simulink model "reference_signal_in_time"  (R2021a)
settings: Solver=VariableStepAuto  StartTime=0.0  StopTime=time_traj(N)+5  RelTol=1e-3
values from neighbouring files (symbols this model uses):
  b = 2    [main_script.m]    (also in trilat2.m = dhat.^2-beacons(:,1).^2-beacons(:,2).^2)
  k1 = 0.5    [main_script.m]
  k1_r = 1    [main_script.m]
  k2 = 1    [main_script.m]
  k2_r = 10    [main_script.m]
  k3_r = 10    [main_script.m]
  N = length(time_traj)    [main_script.m]    (also in trilat2.m = size(beacons,1))
  P0 = diag([0.15 0.15 deg2rad(10)].^2)    [main_script.m]
  S = [  0  100 ... (first row only)    [main_script.m]
  t_sw = time_traj(N-1)+((time_traj(N)-time_traj(N-1))*8/10)    [main_script.m]
  theta0 = 0.001    [main_script.m]
  V = eye(3)*0.01^2    [main_script.m]
  W = 10*diag([1 1 deg2rad(5)].^2)    [main_script.m]
  x0 = x0_g(1,1)+10    [main_script.m]
  x0_g = ginput    [enviroment_plot.m]    (also in main_script.m = enviroment_plot(axis_enviroment))
  y0 = x0_g(1,2)-10    [main_script.m]
libraries: simulink x4, robotcorelib x2
settings Model: Creator=csanc  LastModifiedBy=csanc

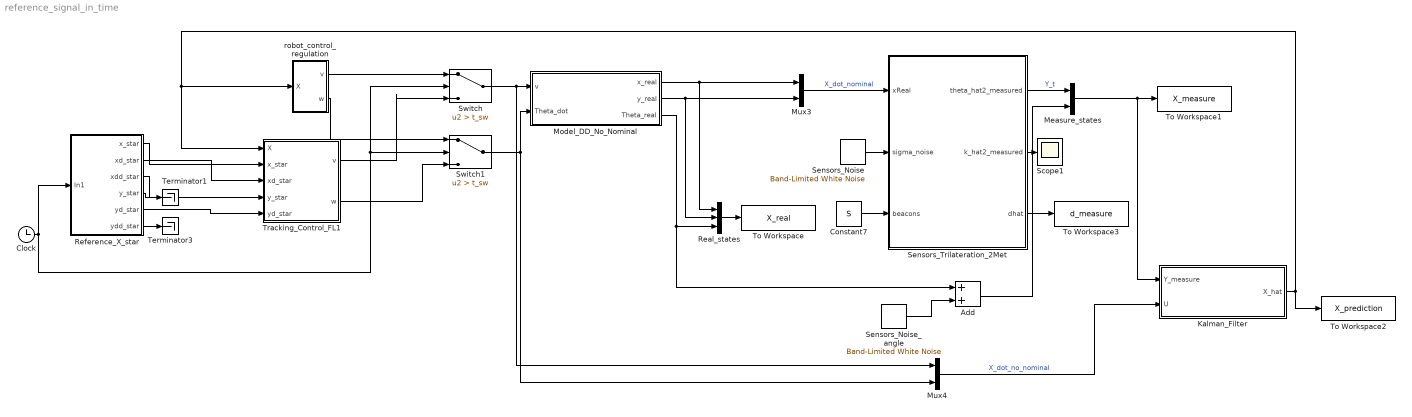
== system reference_signal_in_time ==
  Add : Sum
  Clock : Clock
  Constant7 : Constant  Value=S
  Kalman_Filter : Subsystem
  Measure_states : Mux  Inputs=2
  Model_DD_No_Nominal : Subsystem
  Mux3 : Mux  Inputs=2
  Mux4 : Mux  Inputs=2
  Real_states : Mux  Inputs=3
  Reference_X_star : Subsystem
  Scope1 : Scope
  Sensors_Noise : simulink/Sources/Band-Limited White Noise  Cov=[0.08]  Ts=0.05  seed=[23341]
  Sensors_Noise_angle : simulink/Sources/Band-Limited White Noise  Cov=[0.001]  Ts=0.05  seed=[23341]
  Sensors_Trilateration_2Met : MATLAB Function  TreatAsAtomicUnit=on
  Switch : Switch  Criteria=u2 > Threshold  Threshold=t_sw
  Switch1 : Switch  Criteria=u2 > Threshold  Threshold=t_sw
  Terminator1 : Terminator
  Terminator3 : Terminator
  To Workspace : ToWorkspace  VariableName=X_real  SaveFormat=Structure  SampleTime=-1
  To Workspace1 : ToWorkspace  VariableName=X_measure  SaveFormat=Structure  SampleTime=-1
  To Workspace2 : ToWorkspace  VariableName=X_prediction  SaveFormat=Structure  SampleTime=-1
  To Workspace3 : ToWorkspace  VariableName=d_measure  SaveFormat=Structure  SampleTime=-1
  Tracking_Control_FL1 : Subsystem
  robot_control_regulation : Subsystem
  wires:
  Clock/1 -> Reference_X_star/1(In1), Switch1/2, Switch/2
  Mux4/1 -> Kalman_Filter/2(U)  "X_dot_no_nominal"
  Model_DD_No_Nominal/2(y_real) -> Real_states/2, Mux3/2
  Sensors_Trilateration_2Met/1(theta_hat2_measured) -> Measure_states/1  "Y_t"
  Constant7/1 -> Sensors_Trilateration_2Met/3(beacons)
  Mux3/1 -> Sensors_Trilateration_2Met/1(xReal)  "X_dot_nominal"
  Sensors_Noise/1 -> Sensors_Trilateration_2Met/2(sigma_noise)
  Sensors_Trilateration_2Met/2(k_hat2_measured) -> Scope1/1
  Measure_states/1 -> To Workspace1/1, Kalman_Filter/1(Y_measure)
  Model_DD_No_Nominal/1(x_real) -> Real_states/1, Mux3/1
  Switch/1 -> Mux4/1, Model_DD_No_Nominal/1(v)
  Switch1/1 -> Model_DD_No_Nominal/2(Theta_dot), Mux4/2
  Model_DD_No_Nominal/3(Theta_real) -> Add/1, Real_states/3
  Reference_X_star/3(xdd_star) -> Terminator1/1
  Reference_X_star/6(ydd_star) -> Terminator3/1
  Real_states/1 -> To Workspace/1
  Kalman_Filter/1(X_hat) -> Tracking_Control_FL1/1(X), robot_control_regulation/1(X), To Workspace2/1
  Sensors_Trilateration_2Met/3(dhat) -> To Workspace3/1
  Sensors_Noise_angle/1 -> Add/2
  Add/1 -> Measure_states/2
  robot_control_regulation/1(v) -> Switch/1
  robot_control_regulation/2(w) -> Switch1/1
  Reference_X_star/1(x_star) -> Tracking_Control_FL1/2(x_star)
  Reference_X_star/2(xd_star) -> Tracking_Control_FL1/3(xd_star)
  Reference_X_star/4(y_star) -> Tracking_Control_FL1/4(y_star)
  Reference_X_star/5(yd_star) -> Tracking_Control_FL1/5(yd_star)
  Tracking_Control_FL1/1(v) -> Switch/3
  Tracking_Control_FL1/2(w) -> Switch1/3

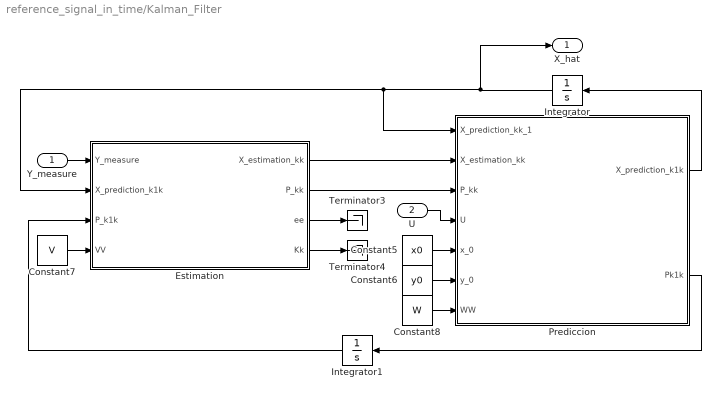
== system reference_signal_in_time/Kalman_Filter ==
  Y_measure : Inport
  U : Inport  Port=2
  Constant5 : Constant  Value=x0
  Constant6 : Constant  Value=y0
  Constant7 : Constant  Value=V
  Constant8 : Constant  Value=W
  Estimation : MATLAB Function  TreatAsAtomicUnit=on
  Integrator : Integrator  InitialCondition=[x0;y0;theta0]
  Integrator1 : Integrator  InitialCondition=P0
  Prediccion : MATLAB Function  TreatAsAtomicUnit=on
  Terminator3 : Terminator
  Terminator4 : Terminator
  X_hat : Outport
  wires:
  Estimation/3(ee) -> Terminator3/1
  Integrator/1 -> X_hat/1, Prediccion/1(X_prediction_kk_1), Estimation/2(X_prediction_k1k)
  Estimation/4(Kk) -> Terminator4/1
  Constant7/1 -> Estimation/4(VV)
  Constant5/1 -> Prediccion/5(x_0)
  Integrator1/1 -> Estimation/3(P_k1k)
  Y_measure/1 -> Estimation/1(Y_measure)
  Constant6/1 -> Prediccion/6(y_0)
  Prediccion/1(X_prediction_k1k) -> Integrator/1
  Prediccion/2(Pk1k) -> Integrator1/1
  Constant8/1 -> Prediccion/7(WW)
  Estimation/1(X_estimation_kk) -> Prediccion/2(X_estimation_kk)
  U/1 -> Prediccion/4(U)
  Estimation/2(P_kk) -> Prediccion/3(P_kk)

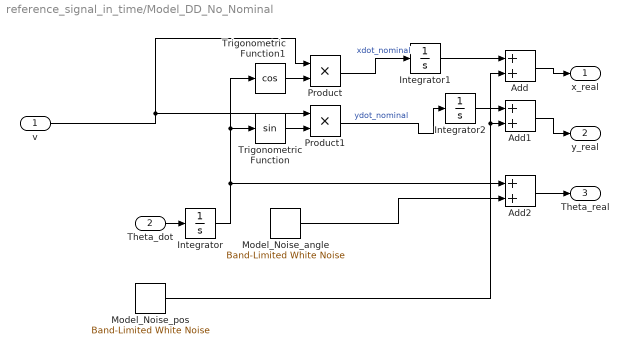
== system reference_signal_in_time/Model_DD_No_Nominal ==
  v : Inport
  Theta_dot : Inport  Port=2
  Add : Sum
  Add1 : Sum
  Add2 : Sum
  Integrator : Integrator  InitialCondition=theta0
  Integrator1 : Integrator  InitialCondition=x0
  Integrator2 : Integrator  InitialCondition=y0
  Model_Noise_angle : simulink/Sources/Band-Limited White Noise  Cov=[0.0001]  Ts=0.05  seed=[23341]
  Model_Noise_pos : simulink/Sources/Band-Limited White Noise  Cov=[0.001]  Ts=0.05  seed=[23341]
  Product : Product
  Product1 : Product
  Trigonometric Function : Trigonometry
  Trigonometric Function1 : Trigonometry  Operator=cos
  x_real : Outport
  y_real : Outport  Port=2
  Theta_real : Outport  Port=3
  wires:
  Theta_dot/1 -> Integrator/1
  Trigonometric Function/1 -> Product1/2
  Product1/1 -> Integrator2/1  "ydot_nominal"
  Trigonometric Function1/1 -> Product/2
  Integrator/1 -> Add2/1, Trigonometric Function/1, Trigonometric Function1/1
  v/1 -> Product/1, Product1/1
  Product/1 -> Integrator1/1  "xdot_nominal"
  Integrator1/1 -> Add/1
  Add/1 -> x_real/1
  Integrator2/1 -> Add1/1
  Add1/1 -> y_real/1
  Add2/1 -> Theta_real/1
  Model_Noise_pos/1 -> Add1/2, Add/2
  Model_Noise_angle/1 -> Add2/2

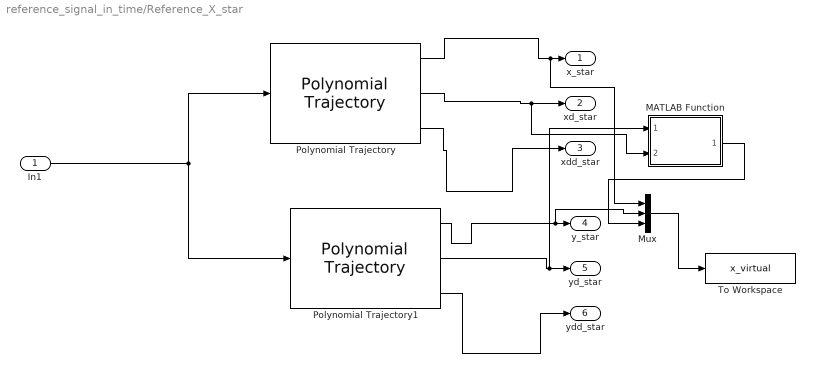
== system reference_signal_in_time/Reference_X_star ==
  In1 : Inport
  MATLAB Function : MATLAB Function  TreatAsAtomicUnit=on
  Mux : Mux  Inputs=3
  Polynomial Trajectory : robotcorelib/Polynomial Trajectory  WaypointSource=Internal  Waypoints=points_x  TimePoints=time_traj  TimeInterval=[ 1, 4 ]  Method=Quintic Polynomial  ParameterSource=Internal  VelocityBoundaryCondition=zeros( 1, N )  AccelerationBoundaryCondition=zeros( 1, N )  SimulateUsing=Interpreted execution
  Polynomial Trajectory1 : robotcorelib/Polynomial Trajectory  WaypointSource=Internal  Waypoints=points_y  TimePoints=time_traj  TimeInterval=[ 1, 4 ]  Method=Quintic Polynomial  ParameterSource=Internal  VelocityBoundaryCondition=zeros( 1, N )  AccelerationBoundaryCondition=zeros( 1, N )  SimulateUsing=Interpreted execution
  To Workspace : ToWorkspace  VariableName=x_virtual  SaveFormat=Structure  SampleTime=-1
  x_star : Outport
  xd_star : Outport  Port=2
  xdd_star : Outport  Port=3
  y_star : Outport  Port=4
  yd_star : Outport  Port=5
  ydd_star : Outport  Port=6
  wires:
  Polynomial Trajectory/1 -> Mux/1, x_star/1
  Polynomial Trajectory/2 -> MATLAB Function/2(x_d_star), xd_star/1
  Polynomial Trajectory/3 -> xdd_star/1
  Polynomial Trajectory1/3 -> ydd_star/1
  Polynomial Trajectory1/2 -> MATLAB Function/1(y_d_star), yd_star/1
  In1/1 -> Polynomial Trajectory/1, Polynomial Trajectory1/1
  Polynomial Trajectory1/1 -> Mux/2, y_star/1
  MATLAB Function/1(Theta_star) -> Mux/3
  Mux/1 -> To Workspace/1

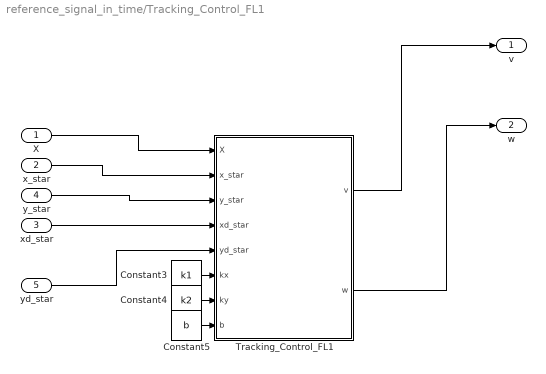
== system reference_signal_in_time/Tracking_Control_FL1 ==
  X : Inport
  x_star : Inport  Port=2
  xd_star : Inport  Port=3
  y_star : Inport  Port=4
  yd_star : Inport  Port=5
  Constant3 : Constant  Value=k1
  Constant4 : Constant  Value=k2
  Constant5 : Constant  Value=b
  Tracking_Control_FL1 : MATLAB Function  TreatAsAtomicUnit=on
  v : Outport
  w : Outport  Port=2
  wires:
  Constant4/1 -> Tracking_Control_FL1/7(ky)
  x_star/1 -> Tracking_Control_FL1/2(x_star)
  Constant5/1 -> Tracking_Control_FL1/8(b)
  Constant3/1 -> Tracking_Control_FL1/6(kx)
  yd_star/1 -> Tracking_Control_FL1/5(yd_star)
  y_star/1 -> Tracking_Control_FL1/3(y_star)
  Tracking_Control_FL1/2(w) -> w/1
  Tracking_Control_FL1/1(v) -> v/1
  xd_star/1 -> Tracking_Control_FL1/4(xd_star)
  X/1 -> Tracking_Control_FL1/1(X)

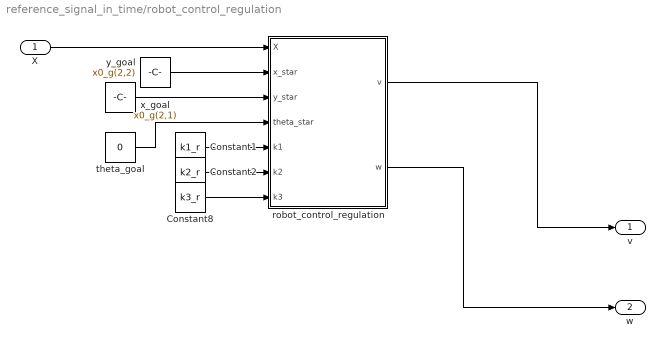
== system reference_signal_in_time/robot_control_regulation ==
  X : Inport
  Constant1 : Constant  Value=k1_r
  Constant2 : Constant  Value=k2_r
  Constant8 : Constant  Value=k3_r
  robot_control_regulation : MATLAB Function  TreatAsAtomicUnit=on
  theta_goal : Constant  Value=0
  x_goal : Constant  Value=x0_g(2,1)
  y_goal : Constant  Value=x0_g(2,2)
  v : Outport
  w : Outport  Port=2
  wires:
  Constant2/1 -> robot_control_regulation/6(k2)
  x_goal/1 -> robot_control_regulation/2(x_star)
  theta_goal/1 -> robot_control_regulation/4(theta_star)
  Constant8/1 -> robot_control_regulation/7(k3)
  robot_control_regulation/1(v) -> v/1
  Constant1/1 -> robot_control_regulation/5(k1)
  y_goal/1 -> robot_control_regulation/3(y_star)
  X/1 -> robot_control_regulation/1(X)
  robot_control_regulation/2(w) -> w/1

== matlab function reference_signal_in_time/Tracking_Control_FL1/Tracking_Control_FL1 ==
  data: v output; X input; x_star input; y_star input; xd_star input; yd_star input; kx input; ky input; b input; w output

function [v,w] = robot_control_for_No_Nominal_FL_sim(X,x_star,y_star,xd_star,yd_star,kx,ky,b)


x=X(1);
y=X(2);
theta=X(3);

xB=x+b*cos(theta);
yB=y+b*sin(theta);

xstar=x_star;
ystar=y_star;

xBdotstar=xd_star;
yBdotstar=yd_star;


Tinv=[
     cos(theta)   sin(theta);
    -sin(theta)/b cos(theta)/b
    ];
ux=xBdotstar+kx*(xstar-xB);
uy=yBdotstar+ky*(ystar-yB);

vw=Tinv*[ux;uy];
v=vw(1);
w=vw(2);
% Xdot=[
%     v*cos(theta);
%     v*sin(theta);
%     w
%     ];

end

== matlab function reference_signal_in_time/robot_control_regulation/robot_control_regulation ==
  data: X input; v output; x_star input; y_star input; theta_star input; k1 input; k2 input; k3 input; w output
function [v,w] = robot_control_regulation(X,x_star,y_star,theta_star,k1,k2,k3)
x=X(1);
y=X(2);
theta=X(3);
% theta_star=atan(y_star/x_star);

ex=x_star-x;
ey=y_star-y;
etheta=delta_angle(theta_star,theta);

rho=norm([ex;ey]);
gamma=delta_angle(atan2(ey,ex),theta);
delta=delta_angle(gamma,etheta);

v=k1*rho*cos(gamma);
w=k2*gamma+k1*(sin(gamma)*cos(gamma)/gamma)*(gamma+k3*delta);


end

== matlab function reference_signal_in_time/Reference_X_star/MATLAB Function ==
  data: y_d_star input; Theta_star output; x_d_star input
function Theta_star = fcn(y_d_star, x_d_star)
Theta_star=atan(y_d_star/x_d_star);

== matlab function reference_signal_in_time/Sensors_Trilateration_2Met ==
  data: theta_hat2_measured output; xReal input; sigma_noise input; beacons input; k_hat2_measured output; dhat output
function [theta_hat2_measured,k_hat2_measured,dhat] = trilateration_second_method(xReal,sigma_noise,beacons)
 
f=@(theta,beacons)(sqrt((beacons(:,1)-theta(1)).^2+(beacons(:,2)-theta(2)).^2));
d=f(xReal,beacons);%distancia entre beacons y medida real
dhat=d+sigma_noise;% distancia con noise de sensor
%% tecnica 2
[theta_hat2_measured,k_hat2_measured]=trilat2(beacons,dhat);

%% Plot
% % figure(4);
% % hold on;
% % grid on;
% % plot(beacons(:,1),beacons(:,2),'ok','LineWidth',3);
% % axis([-5 105 -5 105]);
% % plot(xReal(1),xReal(2),'xb','LineWidth',3);
% % plot(theta_hat2_measured(1),theta_hat2_measured(2),'or','LineWidth',3);
% 
% if enable_real_plot
%     [h]=plot_robot_traj(X',-1,1,[-0.5 1.5 -0.5 1.5]);
% end

== matlab function reference_signal_in_time/Kalman_Filter/Estimation ==
  data: Y_measure input; X_estimation_kk output; X_prediction_k1k input; P_kk output; ee output; Kk output; P_k1k input; VV input
function[X_estimation_kk,P_kk,ee,Kk]=Kalman_Filter(Y_measure,X_prediction_k1k,P_k1k,VV)
Ck=[1 0 0;
    0 1 0
    0 0 1];

%% kalman gain
Kk=P_k1k*Ck'*inv(((Ck*P_k1k*Ck'+VV)));
 %% predicted output
 yhk=Ck*X_prediction_k1k;
%% innovation
ee=Y_measure-yhk;
%% from prediction to estimation
 X_estimation_kk=X_prediction_k1k+Kk*ee;
 P_kk=P_k1k-Kk*Ck*P_k1k;

== matlab function reference_signal_in_time/Kalman_Filter/Prediccion ==
  data: X_prediction_kk_1 input; X_estimation_kk input; X_prediction_k1k output; P_kk input; Pk1k output; U input; x_0 input; y_0 input; WW input
function[X_prediction_k1k, Pk1k]=Kalman_Predictor(X_prediction_kk_1,X_estimation_kk,P_kk,U,x_0,y_0,WW)

theta=atan(X_estimation_kk(2)/X_estimation_kk(1));
A_t=[
    1 0 -U(1)*sin(theta);
    0 1  U(1)*cos(theta);
    0 0             1
    ];
%% from estimation to prediction
X_prediction_k1k=[U(1)*cos(X_prediction_kk_1(3));
    U(1)*sin(X_prediction_kk_1(3));
    U(2)];
Pk1k=A_t.*P_kk.*A_t'+WW;

end
